simulink model "Hierarchical_Control_2018bb"  (R2018b)
settings: Solver=ode45  StartTime=0.0  StopTime=2  RelTol=1e-3
InitFcn:
  | clear all;
  | 
  | Step_time=2;  %并网转离网的切换时间
  | Tf=0.0159*0.25 %直流侧电流滤波常数
  | 
  | Vdc_H2=720;   %直流母线电压最大值
  | Vdc_H1=710;   %
  | Udc=700;   %直流母线电压最大值
  | Vdc_L1=690;
  | Vdc_L2=680;   %直流母线电压最小值
  | 
  | %% 并网变流器部分 %%
  | P_grid=100e3;  %变流器额定功率
  | Cg=3227e-6;   %直流母线电容
  | P_grid=100e3;  %变流器额定功率
  | Idc_max=145;   %直流侧最大输出电流
  | %Rg=(720-700)/Idc_max;   %下垂系数
  | Rg=40*(Udc-40)/P_grid;   %下垂系数
  | Igrid_max=72;   %并网逆变器最大充放电电流（交流侧）
  | 
  | %% 蓄电池部分 %%
  | P_ba=50e3;  %变流器额定功率
  | R_ba=40*(Udc-40)/P_ba;
  | %Idc_max_ba=147;   %直流侧最大输出电流
  | %R_ba=(Vdc_L1-Vdc_L2)/P_ba;   %下垂系数
  | Iba_max=50;   %蓄电池恒流充放电电流
  | 
  | %% 光伏部分 %%
  | P_PV=150e3;  %变流器额定功率
  | R_PV=40*(Udc-40)/P_PV;   %下垂系数
  | Idc_max_PV=147;   %直流侧最大输出电流
undefined symbols (not defined in the file): Ion, Lithium
libraries: powerlib x52, simulink x11, powerlib_meascontrol x9, electricdrivelib x1, re_lib x1
settings Model: SimulationMode=accelerator  Creator=nk123  LastModifiedBy=ZhuanZ
settings SolverCC: AlgebraicLoopSolver=LineSearch
settings OptimizationCC: EfficientMapNaN2IntZero=off
settings HardwareCC: TargetBitPerPointer=64  TargetBitPerSizeT=64  TargetBitPerPtrDiffT=64  TargetLongLongMode=on  TargetIntDivRoundTo=Zero  TargetEndianess=LittleEndian  TargetWordSize=64  TargetHWDeviceType=MATLAB Host  ProdEqTarget=off
settings SFSimCC: SimUseLocalCustomCode=off
settings CodeAppCC: MaxIdLength=128
settings GRTTargetCC: TargetLangStandard=C89/C90 (ANSI)  CombineOutputUpdateFcns=off  GRTInterface=on
settings SimscapeCC: SimscapeNormalizeSystem=off

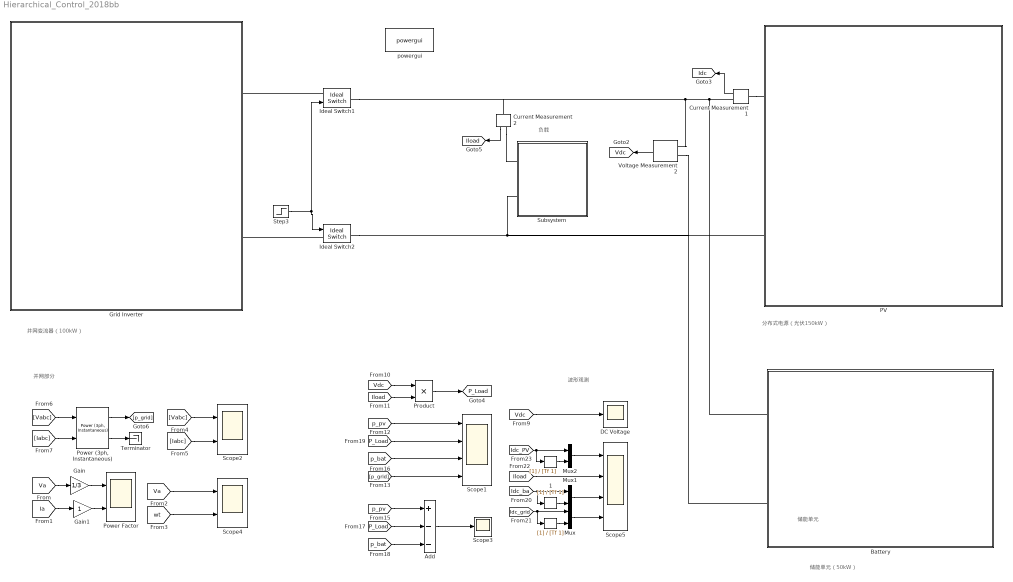
== system Hierarchical_Control_2018bb ==
  note: 波形观测
  note: 储能单元（50kW）
  note: 负载
  note: 并网部分
  note: 并网变流器（100kW）
  note: 分布式电源（光伏150kW）
  note: 储能单元
  " " : TransferFcn  Denominator=[Tf 1]
  "  " : TransferFcn  Denominator=[Tf 1]
  " 1" : TransferFcn  Denominator=[Tf 1]
  Add : Sum  Inputs=+--
  Battery : Subsystem
      mask Display: image(imread('battery.png'))
  Current Measurement1 : powerlib/Measurements/Current Measurement  PhasorSimulation=off  OutputType=Complex  PSBequivalent=0
  Current Measurement2 : powerlib/Measurements/Current Measurement  PhasorSimulation=off  OutputType=Complex  PSBequivalent=0
  DC Voltage : Scope
  Gain : Gain  Gain=1/3
  Gain1 : Gain
  Grid Inverter : Subsystem
      mask Display:
      | disp('并网变流器')
      | image(imread('grid.png'))
  Ideal Switch1 : powerlib/Power Electronics/Ideal Switch  Ron=0.001  Lon=0  IC=1  Rs=1e5  Cs=inf  Measurements=off
  Ideal Switch2 : powerlib/Power Electronics/Ideal Switch  Ron=0.001  Lon=0  IC=1  Rs=1e5  Cs=inf  Measurements=off
  Mux : Mux  Inputs=2
  Mux1 : Mux  Inputs=2
  Mux2 : Mux  Inputs=2
  PV : Subsystem
      mask Display: image(imread('PV.png'))
  "Power (3ph, Instantaneous)" : powerlib_meascontrol/Measurements/Power (3ph, Instantaneous)
      settings: SourceProductName=Simscape Power Systems
  Power Factor : Scope  NumInputPorts=2
  Product : Product
  Scope1 : Scope  NumInputPorts=4
  Scope2 : Scope  NumInputPorts=2
  Scope3 : Scope
  Scope4 : Scope  NumInputPorts=2
  Scope5 : Scope  NumInputPorts=4
  Step3 : Step  Time=Step_time  Before=1  After=0  SampleTime=0
  Subsystem : Subsystem
  Terminator : Terminator
  Voltage Measurement2 : powerlib/Measurements/Voltage Measurement  PhasorSimulation=off  OutputType=Complex  PSBequivalent=0
  powergui : powerlib/powergui  Priority=1  SimulationMode=Discrete  SampleTime=5e-6  frequency=60  Iterations=50  frequencyindice=0  Pbase=100e6  ErrMax=1e-4  UnitsV=kV  UnitsW=MW  buscounter=0  FunctionMessages=off  echomessages=off  EnableUseOfTLC=off  CurrentSourceSwitches=off  DisableSnubberDevices=off  DisableRonSwitches=off  DisableVfSwitches=off  DisplayEquations=off  SolverType=Tustin/Backward Euler (TBE)  Interpol=off  ExternalGateDelay=off  methode=off  Ts=100  x0status=blocks  SPID=on  SwTol=0  HookPort=off  RestoreLinks=warning  ResistiveCurrentMeasurement=off  Frange=[0:2:500]  Ylog=off  Xlog=on  ShowGrid=off  save=off  variable=ZData  structure=0  ZoomFFT=off  StartTime=0.0  cycles=1  DisplayStyle=1  fundamental=60  FreqAxis=off  MaxFrequency=1000  frequencyindicesteady=1  RmsSteady=1  display=off
  tag scope: Idc=global, Iload=global, P_Load=global, Vdc=global
  wires:
  [Iabc] -> Scope2/2
  [Vabc] -> Scope2/1
  [Iabc] -> "Power (3ph, Instantaneous)"/2
  [Vabc] -> "Power (3ph, Instantaneous)"/1
  "Power (3ph, Instantaneous)"/1 -> [p_grid]
  "Power (3ph, Instantaneous)"/2 -> Terminator/1
  [Va] -> Gain/1
  [Ia] -> Gain1/1
  [Va] -> Scope4/1
  [wt] -> Scope4/2
  Voltage Measurement2/1 -> [Vdc]
  [Vdc] -> DC Voltage/1
  Current Measurement1/1 -> [Idc]
  [Iload] -> Product/2
  [Vdc] -> Product/1
  Product/1 -> [P_Load]
  [p_pv] -> Scope1/1
  [P_Load] -> Scope1/2
  [p_pv] -> Add/1
  [P_Load] -> Add/2
  [p_bat] -> Add/3
  Add/1 -> Scope3/1
  [p_bat] -> Scope1/3
  [p_grid] -> Scope1/4
  Current Measurement2/1 -> [Iload]
  Step3/1 -> Ideal Switch2/1, Ideal Switch1/1
  Mux/1 -> Scope5/4
  [Idc_grid] -> " "/1, Mux/1
  Mux2/1 -> Scope5/1
  [Idc_PV] -> "  "/1, Mux2/1
  "  "/1 -> Mux2/2
  [Iload] -> Scope5/2
  Mux1/1 -> Scope5/3
  [Idc_ba] -> " 1"/1, Mux1/1
  " 1"/1 -> Mux1/2
  " "/1 -> Mux/2
  Gain/1 -> Power Factor/1
  Gain1/1 -> Power Factor/2
  connections:
  Battery/LConn2 -- Voltage Measurement2/LConn2 -- PV/LConn2 -- Ideal Switch2/RConn1 -- Subsystem/LConn2
  Current Measurement1/LConn1 -- PV/LConn1
  Battery/LConn1 -- Current Measurement1/RConn1 -- Current Measurement2/LConn1 -- Ideal Switch1/RConn1 -- Voltage Measurement2/LConn1
  Ideal Switch1/LConn1 -- Grid Inverter/LConn1
  Ideal Switch2/LConn1 -- Grid Inverter/LConn2
  Current Measurement2/RConn1 -- Subsystem/LConn1

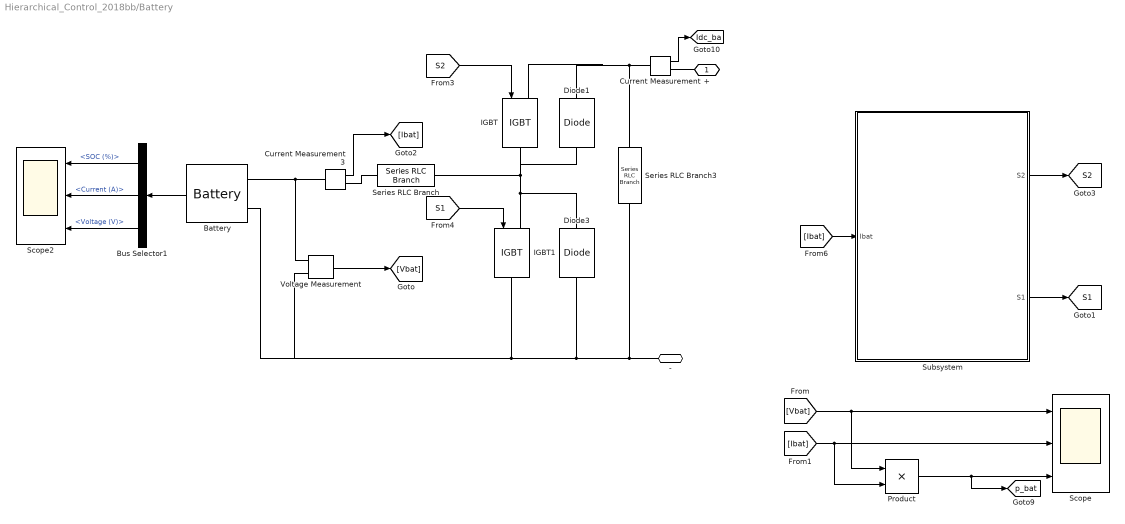
== system Hierarchical_Control_2018bb/Battery ==
  Battery : electricdrivelib/Extra Sources/Battery  BatType=Lithium-Ion  ShowTempParam=off  ThermalPreset=no  ShowAgeParam=off  NomV=300  NomQ=100  SOC=70  Batt_Tr=1  PresetModel=on  MaxQ=100  MinV=225  FullV=349.1961  Dis_rate=43.4783  R=0.03  Normal_OP=90.4348  expZone="[324.1158      4.913043]"  current=[6.5 13 32.5]  Units=Time  Tci=20  NomT=20  T2=-30  MaxQ2=4.8  FullV2=7.1  Normal_OP2=5.655  expZone2="[6.58           1]"  Rca=0.6  ti=2000  Dp=0  Neq0=0  Tsim=1e6  Ta1=25  Qeol=5.4*0.9  Reol=0.013333*1.2  Char_age=[2.3478, 3]  Dis_age=[2.3478, 10]  N1=1500  N2=10500  N3=1000  N4=1400  Ta2=45  N5=950
  Bus Selector1 : BusSelector  OutputSignals=SOC (%),Current (A),Voltage (V)
  Current Measurement : powerlib/Measurements/Current Measurement  PhasorSimulation=off  OutputType=Complex  PSBequivalent=0
  Current Measurement3 : powerlib/Measurements/Current Measurement  PhasorSimulation=off  OutputType=Complex  PSBequivalent=0
  Diode1 : powerlib/Power Electronics/Diode  Ron=0.001  Lon=0  Vf=0.8  IC=0  UseSnubber=off  Rs=500  Cs=250e-9  Measurements=off
  Diode3 : powerlib/Power Electronics/Diode  Ron=0.001  Lon=0  Vf=0.8  IC=0  UseSnubber=off  Rs=500  Cs=250e-9  Measurements=off
  IGBT : powerlib/Power Electronics/IGBT  Ron=0.001  Lon=0  Vf=1  Tf=1e-6  Tt=2e-6  IC=0  Rs=1e5  Cs=inf  Measurements=off
  IGBT1 : powerlib/Power Electronics/IGBT  Ron=0.001  Lon=0  Vf=1  Tf=1e-6  Tt=2e-6  IC=0  Rs=1e5  Cs=inf  Measurements=off
  Product : Product
  Scope : Scope  NumInputPorts=3
  Scope2 : Scope  NumInputPorts=3
  Series RLC Branch : powerlib/Elements/Series RLC Branch  LConnTagsString=__new0  RConnTagsString=__new0  BranchType=L  Resistance=1  Inductance=0.002  SetiL0=off  InitialCurrent=0  Capacitance=1e-6  Setx0=off  InitialVoltage=0  Measurements=None
  Series RLC Branch3 : powerlib/Elements/Series RLC Branch  LConnTagsString=__new0  RConnTagsString=__new0  BranchType=C  Resistance=1  Inductance=1e-3  SetiL0=off  InitialCurrent=0  Capacitance=220e-6  Setx0=off  InitialVoltage=0  Measurements=None
  Subsystem : Subsystem
  Voltage Measurement : powerlib/Measurements/Voltage Measurement  PhasorSimulation=off  OutputType=Complex  PSBequivalent=0
  + : PMIOPort  Side=Left
  - : PMIOPort  Port=2  Side=Left
  tag scope: Idc_ba=global, S1=global, S2=global, p_bat=global
  wires:
  Battery/1 -> Bus Selector1/1
  Bus Selector1/3 -> Scope2/3  "<Voltage (V)>"
  Bus Selector1/1 -> Scope2/1  "<SOC (%)>"
  Bus Selector1/2 -> Scope2/2  "<Current (A)>"
  Voltage Measurement/1 -> [Vbat]
  [Vbat] -> Scope/1, Product/1
  [Ibat] -> Scope/2, Product/2
  Product/1 -> [p_bat], Scope/3
  Current Measurement3/1 -> [Ibat]
  [S1] -> IGBT1/1
  [S2] -> IGBT/1
  Subsystem/1(S2) -> [S2]
  Subsystem/2(S1) -> [S1]
  [Ibat] -> Subsystem/1(Ibat)
  Current Measurement/1 -> [Idc_ba]
  connections:
  Series RLC Branch3/RConn1 -- -/RConn1 -- Diode3/LConn1 -- Voltage Measurement/LConn2 -- Battery/LConn2 -- IGBT1/RConn1
  Series RLC Branch3/LConn1 -- Diode1/RConn1 -- IGBT/LConn1 -- Current Measurement/LConn1
  Voltage Measurement/LConn1 -- Current Measurement3/LConn1 -- Battery/LConn1
  IGBT1/LConn1 -- Series RLC Branch/RConn1 -- Diode1/LConn1 -- IGBT/RConn1 -- Diode3/RConn1
  Current Measurement3/RConn1 -- Series RLC Branch/LConn1
  +/RConn1 -- Current Measurement/RConn1

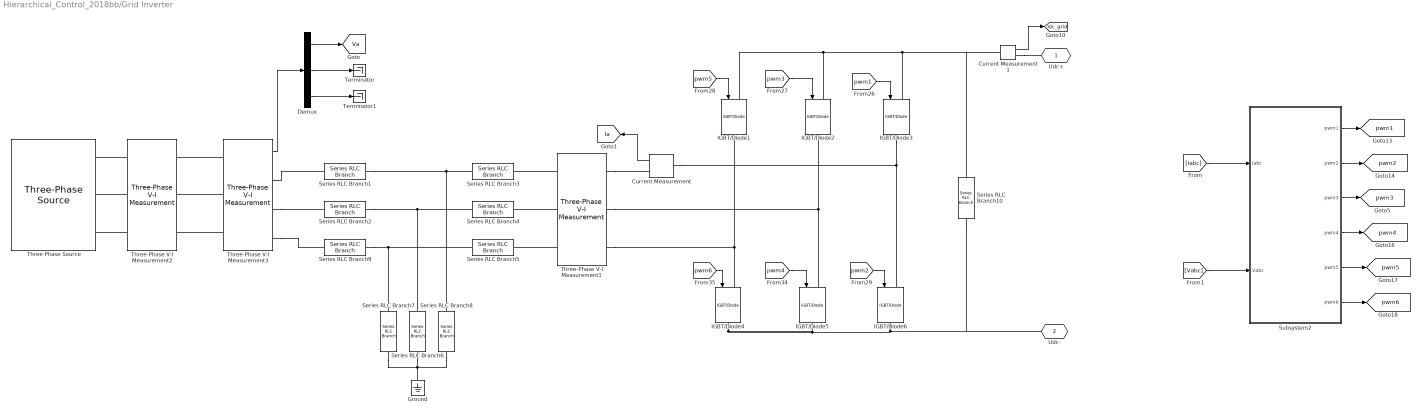
== system Hierarchical_Control_2018bb/Grid Inverter ==
  Current Measurement : powerlib/Measurements/Current Measurement  PhasorSimulation=off  OutputType=Complex  PSBequivalent=0
  Current Measurement1 : powerlib/Measurements/Current Measurement  PhasorSimulation=off  OutputType=Complex  PSBequivalent=0
  Demux : Demux  Outputs=3
  Ground : powerlib/Elements/Ground  LConnTagsString=a
  IGBT/Diode{1..6} (6 alike) : powerlib/Power Electronics/IGBT//Diode  Ron=1e-3  Rs=1e5  Cs=inf  Measurements=off
  Series RLC Branch1 : powerlib/Elements/Series RLC Branch  LConnTagsString=__new0  RConnTagsString=__new0  BranchType=RL  Resistance=1e-3  Inductance=160e-6  SetiL0=off  InitialCurrent=0  Capacitance=1e-6  Setx0=off  InitialVoltage=0  Measurements=None
  Series RLC Branch10 : powerlib/Elements/Series RLC Branch  LConnTagsString=__new0  RConnTagsString=__new0  BranchType=C  Resistance=0.001  Inductance=1e-3  SetiL0=off  InitialCurrent=0  Capacitance=Cg  Setx0=off  InitialVoltage=700  Measurements=None
  Series RLC Branch2 : powerlib/Elements/Series RLC Branch  LConnTagsString=__new0  RConnTagsString=__new0  BranchType=RL  Resistance=1e-3  Inductance=160e-6  SetiL0=off  InitialCurrent=0  Capacitance=1e-6  Setx0=off  InitialVoltage=0  Measurements=None
  Series RLC Branch3 : powerlib/Elements/Series RLC Branch  LConnTagsString=__new0  RConnTagsString=__new0  BranchType=RL  Resistance=1e-3  Inductance=800e-6  SetiL0=off  InitialCurrent=0  Capacitance=1e-6  Setx0=off  InitialVoltage=0  Measurements=None
  Series RLC Branch4 : powerlib/Elements/Series RLC Branch  LConnTagsString=__new0  RConnTagsString=__new0  BranchType=RL  Resistance=1e-3  Inductance=800e-6  SetiL0=off  InitialCurrent=0  Capacitance=1e-6  Setx0=off  InitialVoltage=0  Measurements=None
  Series RLC Branch5 : powerlib/Elements/Series RLC Branch  LConnTagsString=__new0  RConnTagsString=__new0  BranchType=RL  Resistance=1e-3  Inductance=800e-6  SetiL0=off  InitialCurrent=0  Capacitance=1e-6  Setx0=off  InitialVoltage=0  Measurements=None
  Series RLC Branch6 : powerlib/Elements/Series RLC Branch  LConnTagsString=__new0  RConnTagsString=__new0  BranchType=RC  Resistance=1e-3  Inductance=1e-3  SetiL0=off  InitialCurrent=0  Capacitance=109e-6  Setx0=off  InitialVoltage=0  Measurements=None
  Series RLC Branch7 : powerlib/Elements/Series RLC Branch  LConnTagsString=__new0  RConnTagsString=__new0  BranchType=RC  Resistance=1e-3  Inductance=1e-3  SetiL0=off  InitialCurrent=0  Capacitance=109e-6  Setx0=off  InitialVoltage=0  Measurements=None
  Series RLC Branch8 : powerlib/Elements/Series RLC Branch  LConnTagsString=__new0  RConnTagsString=__new0  BranchType=RC  Resistance=1e-3  Inductance=1e-3  SetiL0=off  InitialCurrent=0  Capacitance=109e-6  Setx0=off  InitialVoltage=0  Measurements=None
  Series RLC Branch9 : powerlib/Elements/Series RLC Branch  LConnTagsString=__new0  RConnTagsString=__new0  BranchType=RL  Resistance=1e-3  Inductance=160e-6  SetiL0=off  InitialCurrent=0  Capacitance=1e-6  Setx0=off  InitialVoltage=0  Measurements=None
  Subsystem2 : Subsystem
  Terminator : Terminator
  Terminator1 : Terminator
  Three-Phase V-I Measurement1 : powerlib/Measurements/Three-Phase V-I Measurement  VoltageMeasurement=no  SetLabelV=on  LabelV=Vabc  Vpu=off  VpuLL=off  CurrentMeasurement=yes  SetLabelI=on  LabelI=Iabc  Ipu=off  Pbase=100e6  Vbase=500e3  OutputType=Complex  PhasorSimulation=off  PSBequivalent=0
  Three-Phase V-I Measurement2 : powerlib/Measurements/Three-Phase V-I Measurement  VoltageMeasurement=phase-to-ground  SetLabelV=on  LabelV=Vabc  Vpu=off  VpuLL=off  CurrentMeasurement=no  SetLabelI=on  LabelI=Iabc  Ipu=off  Pbase=100e6  Vbase=500e3  OutputType=Complex  PhasorSimulation=off  PSBequivalent=0
  Three-Phase V-I Measurement3 : powerlib/Measurements/Three-Phase V-I Measurement  VoltageMeasurement=phase-to-ground  SetLabelV=off  LabelV=Vabc  Vpu=off  VpuLL=off  CurrentMeasurement=no  SetLabelI=on  LabelI=Iabc  Ipu=off  Pbase=100e6  Vbase=500e3  OutputType=Complex  PhasorSimulation=off  PSBequivalent=0
  Three-Phase Source : powerlib/Electrical Sources/Three-Phase Source  InternalConnection=Y  VoltagePhases=off  Voltage=380  PhaseAngle=0  Voltage_phases=[25e3 25e3 25e3]/sqrt(3)  PhaseAngles_phases=[0 -120 +120]  Frequency=50  NonIdealSource=on  SpecifyImpedance=off  Resistance=0.001e-3  Inductance=0.001e-9  ShortCircuitLevel=100e6  BaseVoltage=380  XRratio=7  BusType=swing  Pref=10e3  Qref=0  Prefabc=[10e3, 10e3, 10e3]  Qrefabc=[0, 0, 0]  Qmin=-inf  Qmax=inf
  Udc+ : PMIOPort  Side=Left
  Udc- : PMIOPort  Port=2  Side=Left
  tag scope: Ia=global, Idc_grid=global, Va=global, pwm1=global, pwm2=global, pwm3=global, pwm4=global, pwm5=global, pwm6=global
  wires:
  [pwm3] -> IGBT/Diode2/1
  [pwm4] -> IGBT/Diode5/1
  [pwm5] -> IGBT/Diode1/1
  [pwm1] -> IGBT/Diode3/1
  [pwm6] -> IGBT/Diode4/1
  [pwm2] -> IGBT/Diode6/1
  Subsystem2/1(pwm1) -> [pwm1]
  Subsystem2/6(pwm6) -> [pwm6]
  [Iabc] -> Subsystem2/1(Iabc)
  Subsystem2/3(pwm3) -> [pwm3]
  [Vabc] -> Subsystem2/2(Vabc)
  Subsystem2/5(pwm5) -> [pwm5]
  Subsystem2/2(pwm2) -> [pwm2]
  Subsystem2/4(pwm4) -> [pwm4]
  Three-Phase V-I Measurement3/1 -> Demux/1
  Demux/1 -> [Va]
  Current Measurement/1 -> [Ia]
  Demux/2 -> Terminator/1
  Demux/3 -> Terminator1/1
  Current Measurement1/1 -> [Idc_grid]
  connections:
  Series RLC Branch4/RConn1 -- Series RLC Branch2/LConn1 -- Series RLC Branch6/LConn1
  IGBT/Diode4/LConn1 -- Three-Phase V-I Measurement1/LConn3 -- IGBT/Diode1/RConn1
  Series RLC Branch7/RConn1 -- Series RLC Branch8/RConn1 -- Ground/LConn1 -- Series RLC Branch6/RConn1
  IGBT/Diode5/LConn1 -- Three-Phase V-I Measurement1/LConn2 -- IGBT/Diode2/RConn1
  IGBT/Diode3/RConn1 -- IGBT/Diode6/LConn1 -- Current Measurement/LConn1
  IGBT/Diode2/LConn1 -- Series RLC Branch10/LConn1 -- Current Measurement1/LConn1 -- IGBT/Diode3/LConn1 -- IGBT/Diode1/LConn1
  Series RLC Branch7/LConn1 -- Series RLC Branch9/LConn1 -- Series RLC Branch5/RConn1
  Series RLC Branch3/RConn1 -- Series RLC Branch1/LConn1 -- Series RLC Branch8/LConn1
  IGBT/Diode4/RConn1 -- Series RLC Branch10/RConn1 -- Udc-/RConn1 -- IGBT/Diode6/RConn1 -- IGBT/Diode5/RConn1
  Three-Phase V-I Measurement1/RConn1 -- Series RLC Branch3/LConn1
  Three-Phase V-I Measurement1/RConn2 -- Series RLC Branch4/LConn1
  Three-Phase V-I Measurement1/RConn3 -- Series RLC Branch5/LConn1
  Three-Phase V-I Measurement2/LConn3 -- Three-Phase Source/RConn3
  Three-Phase V-I Measurement2/LConn2 -- Three-Phase Source/RConn2
  Three-Phase V-I Measurement2/LConn1 -- Three-Phase Source/RConn1
  Three-Phase V-I Measurement3/LConn1 -- Three-Phase V-I Measurement2/RConn1
  Three-Phase V-I Measurement3/LConn2 -- Three-Phase V-I Measurement2/RConn2
  Three-Phase V-I Measurement3/LConn3 -- Three-Phase V-I Measurement2/RConn3
  Three-Phase V-I Measurement3/RConn1 -- Series RLC Branch1/RConn1
  Three-Phase V-I Measurement3/RConn2 -- Series RLC Branch2/RConn1
  Three-Phase V-I Measurement3/RConn3 -- Series RLC Branch9/RConn1
  Three-Phase V-I Measurement1/LConn1 -- Current Measurement/RConn1
  Current Measurement1/RConn1 -- Udc+/RConn1

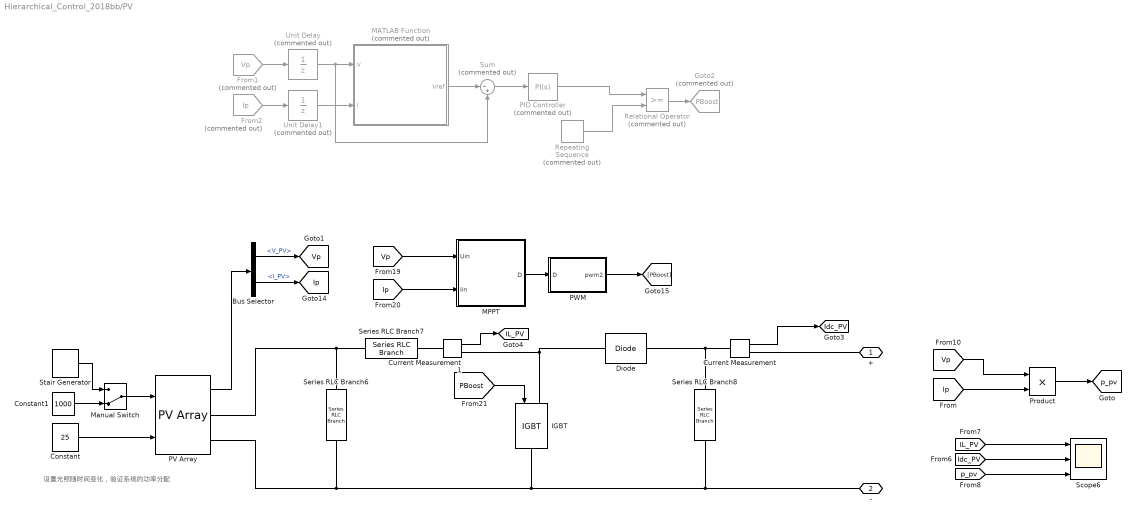
== system Hierarchical_Control_2018bb/PV ==
  note: 设置光照随时间变化，验证系统的功率分配
  Bus Selector : BusSelector  OutputSignals=V_PV,I_PV
  Constant : Constant  Value=25
  Constant1 : Constant  Value=1000
  Current Measurement : powerlib/Measurements/Current Measurement  PhasorSimulation=off  OutputType=Complex  PSBequivalent=0
  Current Measurement1 : powerlib/Measurements/Current Measurement  PhasorSimulation=off  OutputType=Complex  PSBequivalent=0
  Diode : powerlib/Power Electronics/Diode  Ron=0.001  Lon=0  Vf=0.8  IC=0  UseSnubber=off  Rs=500  Cs=250e-9  Measurements=off
  From1 : From  Commented=on  GotoTag=Vp  TagVisibility=global
  From2 : From  Commented=on  GotoTag=Ip  TagVisibility=global
  Goto2 : Goto  Commented=on  GotoTag=PBoost  TagVisibility=global
  IGBT : powerlib/Power Electronics/IGBT  Ron=0.001  Lon=0  Vf=1  Tf=1e-6  Tt=2e-6  IC=0  Rs=1e5  Cs=inf  Measurements=off
  MATLAB Function : MATLAB Function  Commented=on  TreatAsAtomicUnit=on
  MPPT : Subsystem
  Manual Switch : ManualSwitch  CurrentSetting=0
  PID Controller : simulink/Continuous/PID Controller  Commented=on  Controller=PI  Form=Parallel  TimeDomain=Continuous-time  SampleTime=-1  IntegratorMethod=Forward Euler  FilterMethod=Forward Euler  ControllerParametersSource=internal  P=0.005  I=0.001  D=0  UseFilter=on  N=100  TunerSelectOption=Transfer Function Based (PID Tuner App)  InitialConditionSource=internal  InitialConditionForIntegrator=0  InitialConditionForFilter=0  DifferentiatorICPrevScaledInput=0  ExternalReset=none  TrackingMode=off  Kt=1  LimitOutput=on  UpperSaturationLimit=0.95  LowerSaturationLimit=0  LinearizeAsGain=on  AntiWindupMode=none  Kb=1  POutMin=[]  POutMax=[]  IOutMin=[]  IOutMax=[]  DOutMin=[]  DOutMax=[]  NOutMin=[]  NOutMax=[]  SumOutMin=[]  SumOutMax=[]  SaturationOutMin=[]  SaturationOutMax=[]  PParamMin=[]  PParamMax=[]  IParamMin=[]  IParamMax=[]  DParamMin=[]  DParamMax=[]  NParamMin=[]  NParamMax=[]  KbParamMin=[]  KbParamMax=[]  KtParamMin=[]  KtParamMax=[]  KbOutMin=[]  KbOutMax=[]  KtOutMin=[]  KtOutMax=[]  IntegratorOutMin=[]  IntegratorOutMax=[]  FilterOutMin=[]  FilterOutMax=[]  SumI1OutMin=[]  SumI1OutMax=[]  SumI2OutMin=[]  SumI2OutMax=[]  SumI3OutMin=[]  SumI3OutMax=[]  SumI4OutMin=[]  SumI4OutMax=[]  SumDOutMin=[]  SumDOutMax=[]  DifferentiatorOutMin=[]  DifferentiatorOutMax=[]  FilterDiffOutCoefMin=[]  FilterDiffOutCoefMax=[]  ReciprocalOutMin=[]  ReciprocalOutMax=[]  SumDenOutMin=[]  SumDenOutMax=[]  SumNumOutMin=[]  SumNumOutMax=[]  DivideOutMin=[]  DivideOutMax=[]  IntegratorContinuousStateAttributes=''  IntegratorStateMustResolveToSignalObject=off  IntegratorRTWStateStorageClass=Auto  FilterContinuousStateAttributes=''  FilterStateMustResolveToSignalObject=off  FilterRTWStateStorageClass=Auto  ParallelPVariant=InternalParameters  IdealPVariant=Disabled  IVariant=InternalParameters  DVariant=Disabled  IntegratorVariant=Continuous  SatVariant=Enabled  AWVariant=Passthrough  PCopyVariant=Disabled  TRVariant=Disabled  FdbkBlocksVariant=Forward  IdealPFdbkVariant=Disabled  SatFdbkVariant=Disabled  DerivativeFilterVariant=Disabled  NVariant=Disabled  NCopyVariant=Disabled_SignalSpec  FilterICVariant=Disabled  IntegratorICVariant=InternalICs  ExternalResetVariant=Disabled  TRSumVariant=Passthrough  SumFdbkVariant=Disabled  SumVariant=Sum_PI
  PV Array : re_lib/Solar/PV Array  Npar=50  Nser=15  PlotType=array @ 1000 W/m2 & specified temperatures  S_vec="[ 1000  500  100 ]"  Temp_C_vec="[ 45 25  ]"  ModuleName=User-defined  PlotWhenSelected=off  Pm=200  Ncell=60  Voc=36.3  Isc=6.81  Vm=32  Im=6.25  beta_Voc_pc=-0.36099  alpha_Isc_pc=0.102  beta_Voc=-0.13104  alpha_Isc=0.0069462  IL=6.81  I0=1.035e-10  nI=1.0006  Rsh=114.2861  Rs=0.26023  BAL=off  Tc=1e-6  Tfilter=5e-5
  PWM : Subsystem
  Product : Product
  Relational Operator : RelationalOperator  Commented=on  OutDataTypeStr=boolean  RndMeth=Simplest
  Repeating Sequence : simulink/Sources/Repeating Sequence  Commented=on  rep_seq_t=[0 0.0002]  rep_seq_y=[0 1]
  Scope6 : Scope  NumInputPorts=3
  Series RLC Branch6 : powerlib/Elements/Series RLC Branch  LConnTagsString=__new0  RConnTagsString=__new0  BranchType=RC  Resistance=1e-3  Inductance=1e-3  SetiL0=off  InitialCurrent=0  Capacitance=1e-3  Setx0=off  InitialVoltage=0  Measurements=None
  Series RLC Branch7 : powerlib/Elements/Series RLC Branch  LConnTagsString=__new0  RConnTagsString=__new0  BranchType=L  Resistance=1  Inductance=1.45e-3  SetiL0=off  InitialCurrent=0  Capacitance=1e-3  Setx0=off  InitialVoltage=0  Measurements=None
  Series RLC Branch8 : powerlib/Elements/Series RLC Branch  LConnTagsString=__new0  RConnTagsString=__new0  BranchType=C  Resistance=1  Inductance=1e-3  SetiL0=off  InitialCurrent=0  Capacitance=3227e-6  Setx0=off  InitialVoltage=700  Measurements=None
  Stair Generator : powerlib_meascontrol/Pulse & Signal Generators/Stair Generator  t=[0, 0.5, 1, 1.5]  e=[1000, 800, 1200, 800]  Ts=0
      settings: SourceProductName=Simscape Power Systems
  Sum : Sum  Commented=on  Inputs=|-+
  Unit Delay : UnitDelay  Commented=on  SampleTime=1e-4
  Unit Delay1 : UnitDelay  Commented=on  SampleTime=1e-4
  + : PMIOPort  Side=Left
  - : PMIOPort  Port=2  Side=Left
  tag scope: IL_PV=global, Idc_PV=global, Ip=global, Vp=global, p_pv=global
  wires:
  [PBoost] -> IGBT/1
  [Vp] -> Product/1
  Constant/1 -> PV Array/2
  [Ip] -> Product/2
  PV Array/1 -> Bus Selector/1
  Bus Selector/1 -> [Vp]  "<V_PV>"
  Bus Selector/2 -> [Ip]  "<I_PV>"
  [Ip] -> MPPT/2(Iin)
  MPPT/1(D) -> PWM/1(D)
  [Vp] -> MPPT/1(Uin)
  From2/1 -> Unit Delay1/1
  From1/1 -> Unit Delay/1
  Unit Delay/1 -> Sum/2, MATLAB Function/1(V)
  Unit Delay1/1 -> MATLAB Function/2(I)
  MATLAB Function/1(Vref) -> Sum/1
  Sum/1 -> PID Controller/1
  PID Controller/1 -> Relational Operator/1
  Repeating Sequence/1 -> Relational Operator/2
  Relational Operator/1 -> Goto2/1
  Product/1 -> [p_pv]
  Manual Switch/1 -> PV Array/1
  Stair Generator/1 -> Manual Switch/1
  Constant1/1 -> Manual Switch/2
  Current Measurement/1 -> [Idc_PV]
  Current Measurement1/1 -> [IL_PV]
  PWM/1(pwm2) -> [PBoost]
  [IL_PV] -> Scope6/1
  [Idc_PV] -> Scope6/2
  [p_pv] -> Scope6/3
  connections:
  -/RConn1 -- Series RLC Branch8/RConn1 -- IGBT/RConn1 -- Series RLC Branch6/RConn1 -- PV Array/RConn2
  Series RLC Branch6/LConn1 -- Series RLC Branch7/LConn1 -- PV Array/RConn1
  Series RLC Branch8/LConn1 -- Diode/RConn1 -- Current Measurement/LConn1
  IGBT/LConn1 -- Current Measurement1/RConn1 -- Diode/LConn1
  +/RConn1 -- Current Measurement/RConn1
  Current Measurement1/LConn1 -- Series RLC Branch7/RConn1

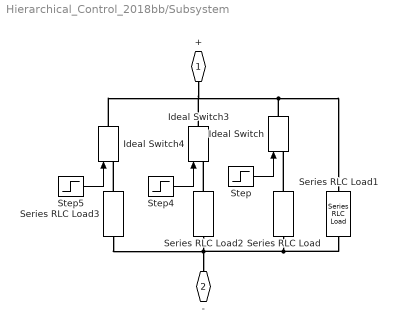
== system Hierarchical_Control_2018bb/Subsystem ==
  Ideal Switch : powerlib/Power Electronics/Ideal Switch  Ron=0.001  Lon=0  IC=0  Rs=1e5  Cs=inf  Measurements=off
  Ideal Switch3 : powerlib/Power Electronics/Ideal Switch  Ron=0.001  Lon=0  IC=0  Rs=1e5  Cs=inf  Measurements=off
  Ideal Switch4 : powerlib/Power Electronics/Ideal Switch  Ron=0.001  Lon=0  IC=0  Rs=1e5  Cs=inf  Measurements=off
  Series RLC Load : powerlib/Elements/Series RLC Load  LConnTagsString=a  RConnTagsString=__new0  NominalVoltage=700  NominalFrequency=50  ActivePower=50e3  InductivePower=0  CapacitivePower=0  Setx0=off  InitialVoltage=0  SetiL0=off  InitialCurrent=0  Measurements=None  LoadType=constant Z
  Series RLC Load1 : powerlib/Elements/Series RLC Load  LConnTagsString=a  RConnTagsString=__new0  NominalVoltage=700  NominalFrequency=50  ActivePower=110e3  InductivePower=0  CapacitivePower=0  Setx0=off  InitialVoltage=0  SetiL0=off  InitialCurrent=0  Measurements=None  LoadType=constant Z
  Series RLC Load2 : powerlib/Elements/Series RLC Load  LConnTagsString=a  RConnTagsString=__new0  NominalVoltage=700  NominalFrequency=50  ActivePower=40e3  InductivePower=0  CapacitivePower=0  Setx0=off  InitialVoltage=0  SetiL0=off  InitialCurrent=0  Measurements=None  LoadType=constant Z
  Series RLC Load3 : powerlib/Elements/Series RLC Load  LConnTagsString=a  RConnTagsString=__new0  NominalVoltage=700  NominalFrequency=50  ActivePower=40e3  InductivePower=0  CapacitivePower=0  Setx0=off  InitialVoltage=0  SetiL0=off  InitialCurrent=0  Measurements=None  LoadType=constant Z
  Step : Step  Time=0.5  SampleTime=0
  Step4 : Step  SampleTime=0
  Step5 : Step  Time=1.5  SampleTime=0
  + : PMIOPort  Side=Left
  - : PMIOPort  Port=2  Side=Left
  wires:
  Step/1 -> Ideal Switch/1
  Step4/1 -> Ideal Switch3/1
  Step5/1 -> Ideal Switch4/1
  connections:
  Series RLC Load2/LConn1 -- Ideal Switch3/LConn1
  Series RLC Load1/RConn1 -- Series RLC Load3/RConn1 -- -/RConn1 -- Series RLC Load2/RConn1 -- Series RLC Load/RConn1
  Ideal Switch/RConn1 -- Ideal Switch4/RConn1 -- +/RConn1 -- Ideal Switch3/RConn1 -- Series RLC Load1/LConn1
  Series RLC Load/LConn1 -- Ideal Switch/LConn1
  Series RLC Load3/LConn1 -- Ideal Switch4/LConn1

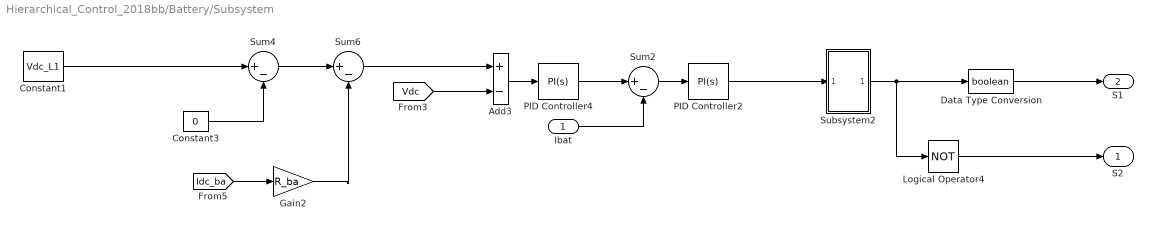
== system Hierarchical_Control_2018bb/Battery/Subsystem ==
  Ibat : Inport
  Add3 : Sum  Inputs=+-
  Constant1 : Constant  Value=Vdc_L1
  Constant3 : Constant  Value=0
  Data Type Conversion : DataTypeConversion  OutDataTypeStr=boolean
  Gain2 : Gain  Gain=R_ba
  Logical Operator4 : Logic  Operator=NOT  AllPortsSameDT=off  OutDataTypeStr=boolean
  PID Controller2 : simulink/Continuous/PID Controller  Controller=PI  Form=Parallel  TimeDomain=Continuous-time  SampleTime=-1  IntegratorMethod=Forward Euler  FilterMethod=Forward Euler  ControllerParametersSource=internal  P=1  I=1  D=0  UseFilter=on  N=100  TunerSelectOption=Transfer Function Based (PID Tuner App)  InitialConditionSource=internal  InitialConditionForIntegrator=0  InitialConditionForFilter=0  DifferentiatorICPrevScaledInput=0  ExternalReset=none  TrackingMode=off  Kt=1  LimitOutput=off  UpperSaturationLimit=inf  LowerSaturationLimit=-inf  LinearizeAsGain=on  AntiWindupMode=none  Kb=1  POutMin=[]  POutMax=[]  IOutMin=[]  IOutMax=[]  DOutMin=[]  DOutMax=[]  NOutMin=[]  NOutMax=[]  SumOutMin=[]  SumOutMax=[]  SaturationOutMin=[]  SaturationOutMax=[]  PParamMin=[]  PParamMax=[]  IParamMin=[]  IParamMax=[]  DParamMin=[]  DParamMax=[]  NParamMin=[]  NParamMax=[]  KbParamMin=[]  KbParamMax=[]  KtParamMin=[]  KtParamMax=[]  KbOutMin=[]  KbOutMax=[]  KtOutMin=[]  KtOutMax=[]  IntegratorOutMin=[]  IntegratorOutMax=[]  FilterOutMin=[]  FilterOutMax=[]  SumI1OutMin=[]  SumI1OutMax=[]  SumI2OutMin=[]  SumI2OutMax=[]  SumI3OutMin=[]  SumI3OutMax=[]  SumI4OutMin=[]  SumI4OutMax=[]  SumDOutMin=[]  SumDOutMax=[]  DifferentiatorOutMin=[]  DifferentiatorOutMax=[]  FilterDiffOutCoefMin=[]  FilterDiffOutCoefMax=[]  ReciprocalOutMin=[]  ReciprocalOutMax=[]  SumDenOutMin=[]  SumDenOutMax=[]  SumNumOutMin=[]  SumNumOutMax=[]  DivideOutMin=[]  DivideOutMax=[]  IntegratorContinuousStateAttributes=''  IntegratorStateMustResolveToSignalObject=off  IntegratorRTWStateStorageClass=Auto  FilterContinuousStateAttributes=''  FilterStateMustResolveToSignalObject=off  FilterRTWStateStorageClass=Auto  ParallelPVariant=InternalParameters  IdealPVariant=Disabled  IVariant=InternalParameters  DVariant=Disabled  IntegratorVariant=Continuous  SatVariant=Disabled  AWVariant=Passthrough  PCopyVariant=Disabled  TRVariant=Disabled  FdbkBlocksVariant=Forward  IdealPFdbkVariant=Disabled  SatFdbkVariant=Disabled  DerivativeFilterVariant=Disabled  NVariant=Disabled  NCopyVariant=Disabled_SignalSpec  FilterICVariant=Disabled  IntegratorICVariant=InternalICs  ExternalResetVariant=Disabled  TRSumVariant=Passthrough  SumFdbkVariant=Disabled  SumVariant=Sum_PI
  PID Controller4 : simulink/Continuous/PID Controller  Controller=PI  Form=Parallel  TimeDomain=Continuous-time  SampleTime=-1  IntegratorMethod=Forward Euler  FilterMethod=Forward Euler  ControllerParametersSource=internal  P=1  I=20  D=0  UseFilter=on  N=100  TunerSelectOption=Transfer Function Based (PID Tuner App)  InitialConditionSource=internal  InitialConditionForIntegrator=0  InitialConditionForFilter=0  DifferentiatorICPrevScaledInput=0  ExternalReset=none  TrackingMode=off  Kt=1  LimitOutput=on  UpperSaturationLimit=Iba_max  LowerSaturationLimit=-Iba_max  LinearizeAsGain=on  AntiWindupMode=none  Kb=1  POutMin=[]  POutMax=[]  IOutMin=[]  IOutMax=[]  DOutMin=[]  DOutMax=[]  NOutMin=[]  NOutMax=[]  SumOutMin=[]  SumOutMax=[]  SaturationOutMin=[]  SaturationOutMax=[]  PParamMin=[]  PParamMax=[]  IParamMin=[]  IParamMax=[]  DParamMin=[]  DParamMax=[]  NParamMin=[]  NParamMax=[]  KbParamMin=[]  KbParamMax=[]  KtParamMin=[]  KtParamMax=[]  KbOutMin=[]  KbOutMax=[]  KtOutMin=[]  KtOutMax=[]  IntegratorOutMin=[]  IntegratorOutMax=[]  FilterOutMin=[]  FilterOutMax=[]  SumI1OutMin=[]  SumI1OutMax=[]  SumI2OutMin=[]  SumI2OutMax=[]  SumI3OutMin=[]  SumI3OutMax=[]  SumI4OutMin=[]  SumI4OutMax=[]  SumDOutMin=[]  SumDOutMax=[]  DifferentiatorOutMin=[]  DifferentiatorOutMax=[]  FilterDiffOutCoefMin=[]  FilterDiffOutCoefMax=[]  ReciprocalOutMin=[]  ReciprocalOutMax=[]  SumDenOutMin=[]  SumDenOutMax=[]  SumNumOutMin=[]  SumNumOutMax=[]  DivideOutMin=[]  DivideOutMax=[]  IntegratorContinuousStateAttributes=''  IntegratorStateMustResolveToSignalObject=off  IntegratorRTWStateStorageClass=Auto  FilterContinuousStateAttributes=''  FilterStateMustResolveToSignalObject=off  FilterRTWStateStorageClass=Auto  ParallelPVariant=InternalParameters  IdealPVariant=Disabled  IVariant=InternalParameters  DVariant=Disabled  IntegratorVariant=Continuous  SatVariant=Enabled  AWVariant=Passthrough  PCopyVariant=Disabled  TRVariant=Disabled  FdbkBlocksVariant=Forward  IdealPFdbkVariant=Disabled  SatFdbkVariant=Disabled  DerivativeFilterVariant=Disabled  NVariant=Disabled  NCopyVariant=Disabled_SignalSpec  FilterICVariant=Disabled  IntegratorICVariant=InternalICs  ExternalResetVariant=Disabled  TRSumVariant=Passthrough  SumFdbkVariant=Disabled  SumVariant=Sum_PI
  Subsystem2 : Subsystem
  Sum2 : Sum  Inputs=|+-
  Sum4 : Sum  Inputs=|+-
  Sum6 : Sum  Inputs=|+-
  S2 : Outport
  S1 : Outport  Port=2
  wires:
  Data Type Conversion/1 -> S1/1
  Ibat/1 -> Sum2/2
  Constant1/1 -> Sum4/1
  Add3/1 -> PID Controller4/1
  Sum4/1 -> Sum6/1
  Gain2/1 -> Sum6/2
  PID Controller2/1 -> Subsystem2/1(In1)
  [Idc_ba] -> Gain2/1
  Sum2/1 -> PID Controller2/1
  [Vdc] -> Add3/2
  Subsystem2/1(Out1) -> Data Type Conversion/1, Logical Operator4/1
  Sum6/1 -> Add3/1
  PID Controller4/1 -> Sum2/1
  Logical Operator4/1 -> S2/1
  Constant3/1 -> Sum4/2

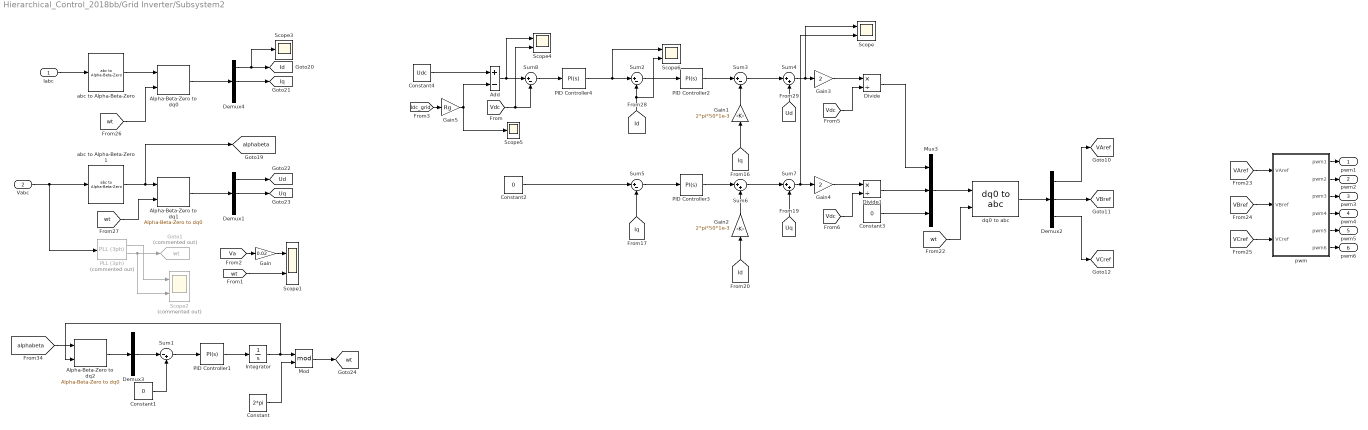
== system Hierarchical_Control_2018bb/Grid Inverter/Subsystem2 ==
  Iabc : Inport
  Vabc : Inport  Port=2
  Add : Sum  Inputs=+-
  Alpha-Beta-Zero to dq0 : powerlib_meascontrol/Transformations/Alpha-Beta-Zero to dq0  Alignment=90 degrees behind phase A axis
      settings: SourceProductName=Simscape Power Systems
  Alpha-Beta-Zero to dq1 : powerlib_meascontrol/Transformations/Alpha-Beta-Zero to dq0  Alignment=90 degrees behind phase A axis
      settings: SourceProductName=Simscape Power Systems
  Alpha-Beta-Zero to dq2 : powerlib_meascontrol/Transformations/Alpha-Beta-Zero to dq0  Alignment=90 degrees behind phase A axis
      settings: SourceProductName=Simscape Power Systems
  Constant : Constant  Value=2*pi
  Constant1 : Constant  Value=0
  Constant2 : Constant  Value=0
  Constant3 : Constant  Value=0
  Constant4 : Constant  Value=Udc
  Demux{1..4} (4 alike) : Demux  Outputs=3
  Divide : Product  Inputs=*/
  Divide1 : Product  Inputs=*/
  Gain : Gain  Gain=0.02
  Gain1 : Gain  Gain=2*pi*50*1e-3
  Gain2 : Gain  Gain=2*pi*50*1e-3
  Gain3 : Gain  Gain=2
  Gain4 : Gain  Gain=2
  Gain5 : Gain  Gain=Rg
  Goto1 : Goto  Commented=on  GotoTag=wt  TagVisibility=global
  Integrator : Integrator
  Mod : Math  Operator=mod  SaturateOnIntegerOverflow=on
  Mux3 : Mux  Inputs=3
  PID Controller1 : simulink/Continuous/PID Controller  Controller=PI  Form=Parallel  TimeDomain=Continuous-time  SampleTime=-1  IntegratorMethod=Forward Euler  FilterMethod=Forward Euler  ControllerParametersSource=internal  P=10  I=50000  D=0  UseFilter=on  N=100  TunerSelectOption=Transfer Function Based (PID Tuner App)  InitialConditionSource=internal  InitialConditionForIntegrator=0  InitialConditionForFilter=0  DifferentiatorICPrevScaledInput=0  ExternalReset=none  TrackingMode=off  Kt=1  LimitOutput=off  UpperSaturationLimit=inf  LowerSaturationLimit=-inf  LinearizeAsGain=on  AntiWindupMode=none  Kb=1  POutMin=[]  POutMax=[]  IOutMin=[]  IOutMax=[]  DOutMin=[]  DOutMax=[]  NOutMin=[]  NOutMax=[]  SumOutMin=[]  SumOutMax=[]  SaturationOutMin=[]  SaturationOutMax=[]  PParamMin=[]  PParamMax=[]  IParamMin=[]  IParamMax=[]  DParamMin=[]  DParamMax=[]  NParamMin=[]  NParamMax=[]  KbParamMin=[]  KbParamMax=[]  KtParamMin=[]  KtParamMax=[]  KbOutMin=[]  KbOutMax=[]  KtOutMin=[]  KtOutMax=[]  IntegratorOutMin=[]  IntegratorOutMax=[]  FilterOutMin=[]  FilterOutMax=[]  SumI1OutMin=[]  SumI1OutMax=[]  SumI2OutMin=[]  SumI2OutMax=[]  SumI3OutMin=[]  SumI3OutMax=[]  SumI4OutMin=[]  SumI4OutMax=[]  SumDOutMin=[]  SumDOutMax=[]  DifferentiatorOutMin=[]  DifferentiatorOutMax=[]  FilterDiffOutCoefMin=[]  FilterDiffOutCoefMax=[]  ReciprocalOutMin=[]  ReciprocalOutMax=[]  SumDenOutMin=[]  SumDenOutMax=[]  SumNumOutMin=[]  SumNumOutMax=[]  DivideOutMin=[]  DivideOutMax=[]  IntegratorContinuousStateAttributes=''  IntegratorStateMustResolveToSignalObject=off  IntegratorRTWStateStorageClass=Auto  FilterContinuousStateAttributes=''  FilterStateMustResolveToSignalObject=off  FilterRTWStateStorageClass=Auto  ParallelPVariant=InternalParameters  IdealPVariant=Disabled  IVariant=InternalParameters  DVariant=Disabled  IntegratorVariant=Continuous  SatVariant=Disabled  AWVariant=Passthrough  PCopyVariant=Disabled  TRVariant=Disabled  FdbkBlocksVariant=Forward  IdealPFdbkVariant=Disabled  SatFdbkVariant=Disabled  DerivativeFilterVariant=Disabled  NVariant=Disabled  NCopyVariant=Disabled_SignalSpec  FilterICVariant=Disabled  IntegratorICVariant=InternalICs  ExternalResetVariant=Disabled  TRSumVariant=Passthrough  SumFdbkVariant=Disabled  SumVariant=Sum_PI
  PID Controller2 : simulink/Continuous/PID Controller  Controller=PI  Form=Parallel  TimeDomain=Continuous-time  SampleTime=-1  IntegratorMethod=Forward Euler  FilterMethod=Forward Euler  ControllerParametersSource=internal  P=10  I=20  D=0  UseFilter=on  N=100  TunerSelectOption=Transfer Function Based (PID Tuner App)  InitialConditionSource=internal  InitialConditionForIntegrator=0  InitialConditionForFilter=0  DifferentiatorICPrevScaledInput=0  ExternalReset=none  TrackingMode=off  Kt=1  LimitOutput=off  UpperSaturationLimit=inf  LowerSaturationLimit=-inf  LinearizeAsGain=on  AntiWindupMode=none  Kb=1  POutMin=[]  POutMax=[]  IOutMin=[]  IOutMax=[]  DOutMin=[]  DOutMax=[]  NOutMin=[]  NOutMax=[]  SumOutMin=[]  SumOutMax=[]  SaturationOutMin=[]  SaturationOutMax=[]  PParamMin=[]  PParamMax=[]  IParamMin=[]  IParamMax=[]  DParamMin=[]  DParamMax=[]  NParamMin=[]  NParamMax=[]  KbParamMin=[]  KbParamMax=[]  KtParamMin=[]  KtParamMax=[]  KbOutMin=[]  KbOutMax=[]  KtOutMin=[]  KtOutMax=[]  IntegratorOutMin=[]  IntegratorOutMax=[]  FilterOutMin=[]  FilterOutMax=[]  SumI1OutMin=[]  SumI1OutMax=[]  SumI2OutMin=[]  SumI2OutMax=[]  SumI3OutMin=[]  SumI3OutMax=[]  SumI4OutMin=[]  SumI4OutMax=[]  SumDOutMin=[]  SumDOutMax=[]  DifferentiatorOutMin=[]  DifferentiatorOutMax=[]  FilterDiffOutCoefMin=[]  FilterDiffOutCoefMax=[]  ReciprocalOutMin=[]  ReciprocalOutMax=[]  SumDenOutMin=[]  SumDenOutMax=[]  SumNumOutMin=[]  SumNumOutMax=[]  DivideOutMin=[]  DivideOutMax=[]  IntegratorContinuousStateAttributes=''  IntegratorStateMustResolveToSignalObject=off  IntegratorRTWStateStorageClass=Auto  FilterContinuousStateAttributes=''  FilterStateMustResolveToSignalObject=off  FilterRTWStateStorageClass=Auto  ParallelPVariant=InternalParameters  IdealPVariant=Disabled  IVariant=InternalParameters  DVariant=Disabled  IntegratorVariant=Continuous  SatVariant=Disabled  AWVariant=Passthrough  PCopyVariant=Disabled  TRVariant=Disabled  FdbkBlocksVariant=Forward  IdealPFdbkVariant=Disabled  SatFdbkVariant=Disabled  DerivativeFilterVariant=Disabled  NVariant=Disabled  NCopyVariant=Disabled_SignalSpec  FilterICVariant=Disabled  IntegratorICVariant=InternalICs  ExternalResetVariant=Disabled  TRSumVariant=Passthrough  SumFdbkVariant=Disabled  SumVariant=Sum_PI
  PID Controller3 : simulink/Continuous/PID Controller  Controller=PI  Form=Parallel  TimeDomain=Continuous-time  SampleTime=-1  IntegratorMethod=Forward Euler  FilterMethod=Forward Euler  ControllerParametersSource=internal  P=10  I=20  D=0  UseFilter=on  N=100  TunerSelectOption=Transfer Function Based (PID Tuner App)  InitialConditionSource=internal  InitialConditionForIntegrator=0  InitialConditionForFilter=0  DifferentiatorICPrevScaledInput=0  ExternalReset=none  TrackingMode=off  Kt=1  LimitOutput=off  UpperSaturationLimit=inf  LowerSaturationLimit=-inf  LinearizeAsGain=on  AntiWindupMode=none  Kb=1  POutMin=[]  POutMax=[]  IOutMin=[]  IOutMax=[]  DOutMin=[]  DOutMax=[]  NOutMin=[]  NOutMax=[]  SumOutMin=[]  SumOutMax=[]  SaturationOutMin=[]  SaturationOutMax=[]  PParamMin=[]  PParamMax=[]  IParamMin=[]  IParamMax=[]  DParamMin=[]  DParamMax=[]  NParamMin=[]  NParamMax=[]  KbParamMin=[]  KbParamMax=[]  KtParamMin=[]  KtParamMax=[]  KbOutMin=[]  KbOutMax=[]  KtOutMin=[]  KtOutMax=[]  IntegratorOutMin=[]  IntegratorOutMax=[]  FilterOutMin=[]  FilterOutMax=[]  SumI1OutMin=[]  SumI1OutMax=[]  SumI2OutMin=[]  SumI2OutMax=[]  SumI3OutMin=[]  SumI3OutMax=[]  SumI4OutMin=[]  SumI4OutMax=[]  SumDOutMin=[]  SumDOutMax=[]  DifferentiatorOutMin=[]  DifferentiatorOutMax=[]  FilterDiffOutCoefMin=[]  FilterDiffOutCoefMax=[]  ReciprocalOutMin=[]  ReciprocalOutMax=[]  SumDenOutMin=[]  SumDenOutMax=[]  SumNumOutMin=[]  SumNumOutMax=[]  DivideOutMin=[]  DivideOutMax=[]  IntegratorContinuousStateAttributes=''  IntegratorStateMustResolveToSignalObject=off  IntegratorRTWStateStorageClass=Auto  FilterContinuousStateAttributes=''  FilterStateMustResolveToSignalObject=off  FilterRTWStateStorageClass=Auto  ParallelPVariant=InternalParameters  IdealPVariant=Disabled  IVariant=InternalParameters  DVariant=Disabled  IntegratorVariant=Continuous  SatVariant=Disabled  AWVariant=Passthrough  PCopyVariant=Disabled  TRVariant=Disabled  FdbkBlocksVariant=Forward  IdealPFdbkVariant=Disabled  SatFdbkVariant=Disabled  DerivativeFilterVariant=Disabled  NVariant=Disabled  NCopyVariant=Disabled_SignalSpec  FilterICVariant=Disabled  IntegratorICVariant=InternalICs  ExternalResetVariant=Disabled  TRSumVariant=Passthrough  SumFdbkVariant=Disabled  SumVariant=Sum_PI
  PID Controller4 : simulink/Continuous/PID Controller  Controller=PI  Form=Parallel  TimeDomain=Continuous-time  SampleTime=-1  IntegratorMethod=Forward Euler  FilterMethod=Forward Euler  ControllerParametersSource=internal  P=0.25  I=30  D=0  UseFilter=on  N=100  TunerSelectOption=Transfer Function Based (PID Tuner App)  InitialConditionSource=internal  InitialConditionForIntegrator=0  InitialConditionForFilter=0  DifferentiatorICPrevScaledInput=0  ExternalReset=none  TrackingMode=off  Kt=1  LimitOutput=on  UpperSaturationLimit=Igrid_max  LowerSaturationLimit=-Igrid_max  LinearizeAsGain=on  AntiWindupMode=none  Kb=1  POutMin=[]  POutMax=[]  IOutMin=[]  IOutMax=[]  DOutMin=[]  DOutMax=[]  NOutMin=[]  NOutMax=[]  SumOutMin=[]  SumOutMax=[]  SaturationOutMin=[]  SaturationOutMax=[]  PParamMin=[]  PParamMax=[]  IParamMin=[]  IParamMax=[]  DParamMin=[]  DParamMax=[]  NParamMin=[]  NParamMax=[]  KbParamMin=[]  KbParamMax=[]  KtParamMin=[]  KtParamMax=[]  KbOutMin=[]  KbOutMax=[]  KtOutMin=[]  KtOutMax=[]  IntegratorOutMin=[]  IntegratorOutMax=[]  FilterOutMin=[]  FilterOutMax=[]  SumI1OutMin=[]  SumI1OutMax=[]  SumI2OutMin=[]  SumI2OutMax=[]  SumI3OutMin=[]  SumI3OutMax=[]  SumI4OutMin=[]  SumI4OutMax=[]  SumDOutMin=[]  SumDOutMax=[]  DifferentiatorOutMin=[]  DifferentiatorOutMax=[]  FilterDiffOutCoefMin=[]  FilterDiffOutCoefMax=[]  ReciprocalOutMin=[]  ReciprocalOutMax=[]  SumDenOutMin=[]  SumDenOutMax=[]  SumNumOutMin=[]  SumNumOutMax=[]  DivideOutMin=[]  DivideOutMax=[]  IntegratorContinuousStateAttributes=''  IntegratorStateMustResolveToSignalObject=off  IntegratorRTWStateStorageClass=Auto  FilterContinuousStateAttributes=''  FilterStateMustResolveToSignalObject=off  FilterRTWStateStorageClass=Auto  ParallelPVariant=InternalParameters  IdealPVariant=Disabled  IVariant=InternalParameters  DVariant=Disabled  IntegratorVariant=Continuous  SatVariant=Enabled  AWVariant=Passthrough  PCopyVariant=Disabled  TRVariant=Disabled  FdbkBlocksVariant=Forward  IdealPFdbkVariant=Disabled  SatFdbkVariant=Disabled  DerivativeFilterVariant=Disabled  NVariant=Disabled  NCopyVariant=Disabled_SignalSpec  FilterICVariant=Disabled  IntegratorICVariant=InternalICs  ExternalResetVariant=Disabled  TRSumVariant=Passthrough  SumFdbkVariant=Disabled  SumVariant=Sum_PI
  PLL (3ph) : powerlib_meascontrol/PLL/PLL (3ph)  Commented=on  Fmin=45  Par_Init=[0, 60]  ParK=[10, 50000, 1]  TcD=1e-4  MaxRateChangeFreq=12  FilterCutOffFreq=25  Ts=0  AGC=on
  Scope{,1,4,6} (4 alike) : Scope  NumInputPorts=2
  Scope2 : Scope  Commented=on  NumInputPorts=2
  Scope3 : Scope
  Scope5 : Scope
  Sum1 : Sum  Inputs=|-+
  Sum{2..3,5,8} (4 alike) : Sum  Inputs=|+-
  Sum4 : Sum  Inputs=|++
  Sum6 : Sum  Inputs=|++
  Sum7 : Sum  Inputs=|++
  abc to Alpha-Beta-Zero : powerlib_meascontrol/Transformations/abc to Alpha-Beta-Zero
      settings: SourceProductName=Simscape Power Systems
  abc to Alpha-Beta-Zero1 : powerlib_meascontrol/Transformations/abc to Alpha-Beta-Zero
      settings: SourceProductName=Simscape Power Systems
  dq0 to abc : powerlib_meascontrol/Transformations/dq0 to abc  Alignment=90 degrees behind phase A axis
  pwm : Subsystem
  pwm1 : Outport
  pwm2 : Outport  Port=2
  pwm3 : Outport  Port=3
  pwm4 : Outport  Port=4
  pwm5 : Outport  Port=5
  pwm6 : Outport  Port=6
  tag scope: Id=global, Iq=global, Ud=global, Uq=global, VAref=global, VBref=global, VCref=global, alphabeta=global, wt=global
  wires:
  [VBref] -> pwm/2(VBref)
  Alpha-Beta-Zero to dq2/1 -> Demux3/1
  Sum1/1 -> PID Controller1/1
  PID Controller2/1 -> Sum3/1
  Constant2/1 -> Sum5/1
  Gain1/1 -> Sum3/2
  Sum2/1 -> PID Controller2/1
  [Id] -> Gain2/1
  Demux2/2 -> [VBref]
  pwm/5(pwm5) -> pwm5/1
  [VAref] -> pwm/1(VAref)
  Alpha-Beta-Zero to dq1/1 -> Demux1/1
  PID Controller1/1 -> Integrator/1
  Alpha-Beta-Zero to dq0/1 -> Demux4/1
  [Iq] -> Sum5/2
  [wt] -> Alpha-Beta-Zero to dq0/2
  PID Controller3/1 -> Sum6/1
  [Uq] -> Sum7/2
  pwm/6(pwm6) -> pwm6/1
  dq0 to abc/1 -> Demux2/1
  [Ud] -> Sum4/2
  Demux1/2 -> [Uq]
  Gain2/1 -> Sum6/2
  Sum3/1 -> Sum4/1
  Demux1/1 -> [Ud]
  Demux4/1 -> Scope3/1, [Id]
  abc to Alpha-Beta-Zero1/1 -> [alphabeta], Alpha-Beta-Zero to dq1/1
  Mux3/1 -> dq0 to abc/1
  pwm/2(pwm2) -> pwm2/1
  abc to Alpha-Beta-Zero/1 -> Alpha-Beta-Zero to dq0/1
  [Iq] -> Gain1/1
  Demux4/2 -> [Iq]
  Sum5/1 -> PID Controller3/1
  Sum6/1 -> Sum7/1
  pwm/1(pwm1) -> pwm1/1
  Demux2/1 -> [VAref]
  Integrator/1 -> Mod/1, Alpha-Beta-Zero to dq2/2
  [Id] -> Scope6/2, Sum2/2
  Demux2/3 -> [VCref]
  [alphabeta] -> Alpha-Beta-Zero to dq2/1
  [wt] -> Alpha-Beta-Zero to dq1/2
  [VCref] -> pwm/3(VCref)
  pwm/3(pwm3) -> pwm3/1
  pwm/4(pwm4) -> pwm4/1
  Constant4/1 -> Add/1
  Demux3/2 -> Sum1/1
  Constant1/1 -> Sum1/2
  Gain3/1 -> Divide/1
  [Vdc] -> Divide/2
  [Vdc] -> Divide1/2
  Gain4/1 -> Divide1/1
  Sum7/1 -> Scope/2, Gain4/1
  Divide1/1 -> Mux3/2
  Divide/1 -> Mux3/1
  [wt] -> dq0 to abc/2
  Iabc/1 -> abc to Alpha-Beta-Zero/1
  Sum4/1 -> Scope/1, Gain3/1
  Mod/1 -> [wt]
  Constant/1 -> Mod/2
  [wt] -> Scope1/2
  [Va] -> Gain/1
  Gain/1 -> Scope1/1
  PLL (3ph)/2 -> Scope2/2, Goto1/1
  PLL (3ph)/1 -> Scope2/1
  Vabc/1 -> PLL (3ph)/1, abc to Alpha-Beta-Zero1/1
  Constant3/1 -> Mux3/3
  [Idc_grid] -> Gain5/1
  PID Controller4/1 -> Scope6/1, Sum2/1
  Gain5/1 -> Scope5/1, Add/2
  Add/1 -> Sum8/1, Scope4/1
  Sum8/1 -> PID Controller4/1
  [Vdc] -> Sum8/2, Scope4/2

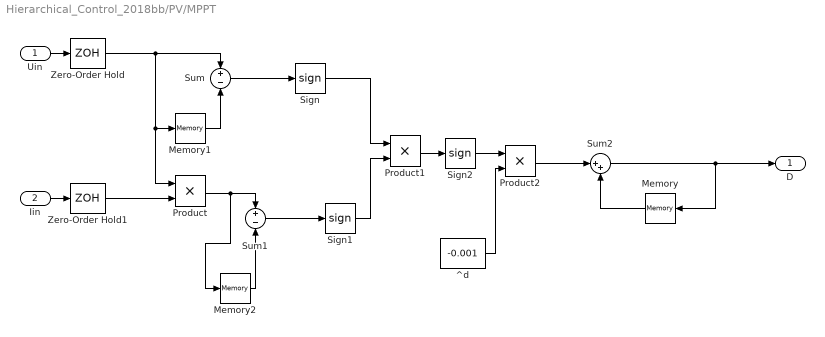
== system Hierarchical_Control_2018bb/PV/MPPT ==
  Uin : Inport
  Iin : Inport  Port=2
  Memory : Memory  InitialCondition=0.85
  Memory1 : Memory  InitialCondition=0.5
  Memory2 : Memory  InitialCondition=10
  Product : Product  RndMeth=Zero
  Product1 : Product  RndMeth=Zero
  Product2 : Product  RndMeth=Zero
  Sign : Signum  SampleTime=0
  Sign1 : Signum  SampleTime=0
  Sign2 : Signum
  Sum : Sum  Inputs=+-
  Sum1 : Sum  Inputs=+-
  Sum2 : Sum  Inputs=|++
  Zero-Order Hold : ZeroOrderHold  SampleTime=1e-4
  Zero-Order Hold1 : ZeroOrderHold  SampleTime=1e-4
  ^d : Constant  Value=-0.001
  D : Outport
  wires:
  Zero-Order Hold/1 -> Sum/1, Memory1/1, Product/1
  Sum/1 -> Sign/1
  Memory1/1 -> Sum/2
  Zero-Order Hold1/1 -> Product/2
  Product/1 -> Sum1/1, Memory2/1
  Sum1/1 -> Sign1/1
  Memory2/1 -> Sum1/2
  Sign1/1 -> Product1/2
  Sign/1 -> Product1/1
  ^d/1 -> Product2/2
  Sum2/1 -> Memory/1, D/1
  Memory/1 -> Sum2/2
  Uin/1 -> Zero-Order Hold/1
  Iin/1 -> Zero-Order Hold1/1
  Sign2/1 -> Product2/1
  Product1/1 -> Sign2/1
  Product2/1 -> Sum2/1

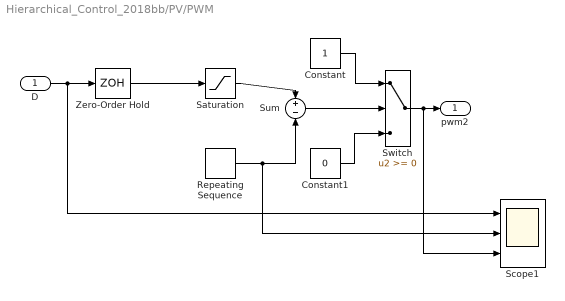
== system Hierarchical_Control_2018bb/PV/PWM ==
  D : Inport
  Constant : Constant
  Constant1 : Constant  Value=0
  Repeating Sequence : simulink/Sources/Repeating Sequence  rep_seq_t=[0 1e-4]  rep_seq_y=[0 1]
  Saturation : Saturate  UpperLimit=1  LowerLimit=-1  SampleTime=0
  Scope1 : Scope  NumInputPorts=3
  Sum : Sum  Inputs=+-
  Switch : Switch
  Zero-Order Hold : ZeroOrderHold  SampleTime=1e-4
  pwm2 : Outport
  wires:
  D/1 -> Scope1/1, Zero-Order Hold/1
  Zero-Order Hold/1 -> Saturation/1
  Saturation/1 -> Sum/1
  Repeating Sequence/1 -> Scope1/2, Sum/2
  Sum/1 -> Switch/2
  Constant/1 -> Switch/1
  Constant1/1 -> Switch/3
  Switch/1 -> Scope1/3, pwm2/1

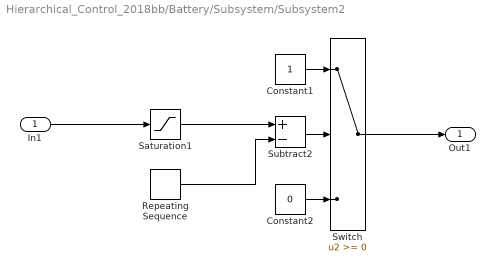
== system Hierarchical_Control_2018bb/Battery/Subsystem/Subsystem2 ==
  In1 : Inport
  Constant1 : Constant
  Constant2 : Constant  Value=0
  Repeating Sequence : simulink/Sources/Repeating Sequence  rep_seq_t=[0 0.00005 0.0001]  rep_seq_y=[-1 1 -1]
  Saturation1 : Saturate  UpperLimit=1  LowerLimit=-1
  Subtract2 : Sum  Inputs=+-
  Switch : Switch
  Out1 : Outport
  wires:
  Switch/1 -> Out1/1
  Constant2/1 -> Switch/3
  Constant1/1 -> Switch/1
  Repeating Sequence/1 -> Subtract2/2
  Subtract2/1 -> Switch/2
  Saturation1/1 -> Subtract2/1
  In1/1 -> Saturation1/1

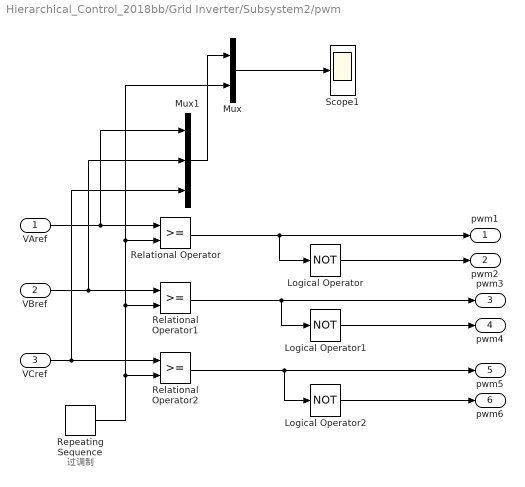
== system Hierarchical_Control_2018bb/Grid Inverter/Subsystem2/pwm ==
  note: 过调制
  VAref : Inport
  VBref : Inport  Port=2
  VCref : Inport  Port=3
  Logical Operator : Logic  Operator=NOT  AllPortsSameDT=off  OutDataTypeStr=boolean
  Logical Operator1 : Logic  Operator=NOT  AllPortsSameDT=off  OutDataTypeStr=boolean
  Logical Operator2 : Logic  Operator=NOT  AllPortsSameDT=off  OutDataTypeStr=boolean
  Mux : Mux  Inputs=2
  Mux1 : Mux  Inputs=3
  Relational Operator : RelationalOperator  OutDataTypeStr=boolean  RndMeth=Simplest
  Relational Operator1 : RelationalOperator  OutDataTypeStr=boolean  RndMeth=Simplest
  Relational Operator2 : RelationalOperator  OutDataTypeStr=boolean  RndMeth=Simplest
  Repeating Sequence : simulink/Sources/Repeating Sequence  rep_seq_t=[0 0.00005 0.0001]  rep_seq_y=[-1 1 -1]
  Scope1 : Scope
  pwm1 : Outport
  pwm2 : Outport  Port=2
  pwm3 : Outport  Port=3
  pwm4 : Outport  Port=4
  pwm5 : Outport  Port=5
  pwm6 : Outport  Port=6
  wires:
  Repeating Sequence/1 -> Relational Operator2/2, Relational Operator1/2, Mux/2, Relational Operator/2
  VCref/1 -> Mux1/3, Relational Operator2/1
  Logical Operator1/1 -> pwm4/1
  Relational Operator/1 -> pwm1/1, Logical Operator/1
  Relational Operator1/1 -> pwm3/1, Logical Operator1/1
  Logical Operator2/1 -> pwm6/1
  VBref/1 -> Mux1/2, Relational Operator1/1
  Relational Operator2/1 -> pwm5/1, Logical Operator2/1
  VAref/1 -> Mux1/1, Relational Operator/1
  Logical Operator/1 -> pwm2/1
  Mux/1 -> Scope1/1
  Mux1/1 -> Mux/1

== matlab function Hierarchical_Control_2018bb/PV/MATLAB Function ==
  data: V input; Vref output; I input
function Vref =RefGen(V, I)

Vrefmax = 363;
Vrefmin = 0.0;
Vrefinit= 300;
deltaVref = 1;
persistent Vold Pold Vrefold;

dataType = 'double';

if isempty(Vold)
    Vold=0;
    Pold=0;
    Vrefold=Vrefinit;
end
P= V*I;
dV=V-Vold;
dP=P-Pold;

if dP ~=0;
    if dP<0
        if dV<0
            Vref=Vrefold +deltaVref;
        else
            Vref=Vrefold -deltaVref;
        end
    else
        if dV<0
            Vref=Vrefold -deltaVref;
        else
            Vref=Vrefold +deltaVref;
        end 
    end
else Vref=Vrefold
end

if Vref>= Vrefmax | Vref<=Vrefmin
    Vref=Vrefold;
end

Vrefold=Vref;
Vold=V;
Pold=P;
